simulink model "MPC"  (R2022b)
settings: Solver=VariableStepAuto  StartTime=0.0  StopTime=T_final*2  RelTol=1e-3
values from neighbouring files (symbols this model uses):
  Aineq = [zeros(n_int*L,n_states*(L+1)) eye(n_int*L) -eye(n_int*L) ... (first row only)    [Run_model.m]
  bineq = [kron(ones(L,1),u_up) ... (first row only)    [Run_model.m]
  d = 0.1    [Run_model.m]
  H = blkdiag(H1,H2,H3)    [Run_model.m]
  L = 10    [Run_model.m]    (also in encoder.m = 0.1175; measurement_model.m = 0.1175)
  n_int = 2    [Run_model.m]
  n_states = 3    [Run_model.m]
  Ts = 0.01    [Run_model.m]    (also in imu.m)
  z_initial = [theta0;x0;y0]    [Run_model.m]
settings Model: Creator=Abelb  LastModifiedBy=Abelb

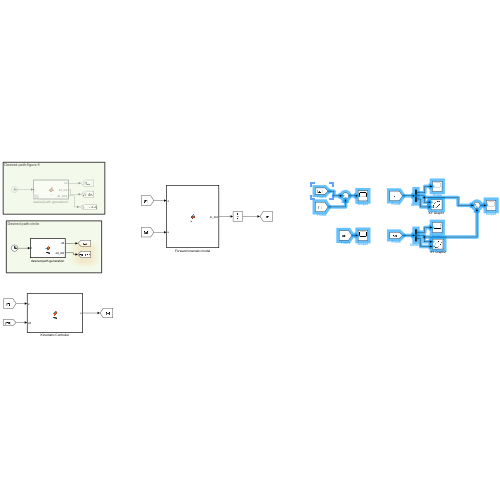
[thumbnail: Simulink's stored preview of the top-level diagram]
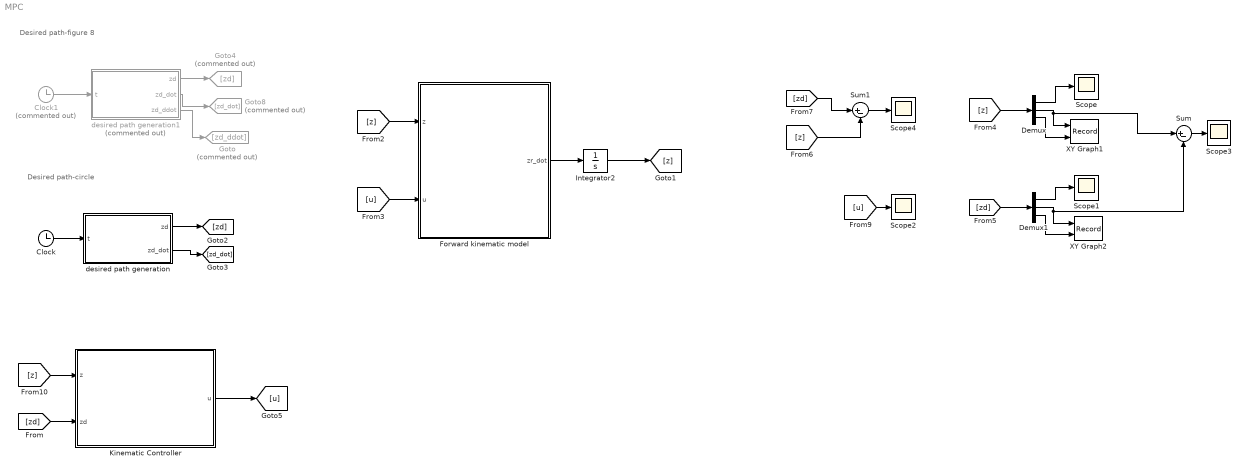
== system MPC ==
  note: Desired path-circle
  note: Desired path-figure 8
  Clock : Clock
  Clock1 : Clock  Commented=on
  Demux : Demux  Outputs=3
  Demux1 : Demux  Outputs=3
  Forward kinematic model : MATLAB Function  TreatAsAtomicUnit=on
  Goto : Goto  Commented=on  GotoTag=zd_ddot
  Goto4 : Goto  Commented=on  GotoTag=zd
  Goto8 : Goto  Commented=on  GotoTag=zd_dot
  Integrator2 : Integrator  InitialCondition=z_initial
  Kinematic Controller : MATLAB Function  TreatAsAtomicUnit=on
  Scope{,1..4} (5 alike) : Scope
  Sum : Sum  Inputs=|+-
  Sum1 : Sum  Inputs=|+-
  XY Graph1 : Record  FileSettingsInternal="{\"entries\":[{\"content\":{\"excelSettings\":{\"content\":{},\"type\":\"Streamout.ExcelSettings\"}},\"type\":\"Streamout.FileSettingStorage\",\"uuid\":\"ce67c0c4-7f67-4c88-aaae-392a4bc8995e\"}],\"packageUris\":[\"http://schema.mathworks.com/mf0/streamout_blocks/R2020a\"],\"version\":\"1.0\"}"  Layout=[1 1]  SignalsInternal="{\"entries\":[{\"content\":{\"signals\":[{\"content\":{\"blockPath\":[\"MPC/XY Graph1\"],\"channel\":[],\"dimensions\":[1],\"domain\":\"MPC/XY Graph1\",\"lineColor\":\"#a2142f\",\"plots\":[1],\"port\":1,\"sid\":[\"\"],\"signalID\":31603,\"signalName\":\"Demux:2\"},\"type\":\"RecordBlkView.Signal\",\"uuid\":\"af874ebe-007b-4861-a05c-edfc673b51a8\"},{\"content\":{\"blockPath\":[\"MPC/XY Graph1\"],\"channel\":[],\"dimensions\":[1],\"domain\":\"MPC/XY Graph1\",\"lineColor\":\"#139fff\",\"plots\":[1],\"port\":2,\"sid\":[\"\"],\"signalID\":31607,\"signalName\":\"Demux:3\"},\"type\":\"RecordBlkView.Signal\",\"uuid\":\"9c7c2835-5321-4135-b8aa-964658d863e7\"}]},\"type\":\"RecordBlkView.InputSignals\",\"uuid\":\"460cb3ef-f7a3-4bdc-882a-30f64cb38d6e\"}],\"packageUris\":[\"http://schema.mathworks.com/mf0/streamout_blocks/R2020a\"],\"version\":\"1.0\"}"  VisualizationBindings="{\"xyplotplugin\":{\"info\":[{\"series\":[{\"bindingParametersList\":[{\"parameter\":\"X-Axis\",\"signalID\":31603,\"signalName\":\"Demux:2\"},{\"parameter\":\"Y-Axis\",\"signalID\":31607,\"signalName\":\"Demux:3\"}],\"seriesID\":48364}],\"subplotID\":1}]}}"  CompatibilityTag=XY
  XY Graph2 : Record  FileSettingsInternal="{\"entries\":[{\"content\":{\"excelSettings\":{\"content\":{},\"type\":\"Streamout.ExcelSettings\"}},\"type\":\"Streamout.FileSettingStorage\",\"uuid\":\"94404df9-d188-4410-a8ad-29bdb399ae23\"}],\"packageUris\":[\"http://schema.mathworks.com/mf0/streamout_blocks/R2020a\"],\"version\":\"1.0\"}"  Layout=[1 1]  SignalsInternal="{\"entries\":[{\"content\":{\"signals\":[{\"content\":{\"blockPath\":[\"MPC/XY Graph2\"],\"channel\":[],\"dimensions\":[1],\"domain\":\"MPC/XY Graph2\",\"lineColor\":\"#a2142f\",\"plots\":[1],\"port\":1,\"sid\":[\"\"],\"signalID\":31611,\"signalName\":\"Demux1:2\"},\"type\":\"RecordBlkView.Signal\",\"uuid\":\"86dd43ab-7c69-451e-8692-9ec7fed00778\"},{\"content\":{\"blockPath\":[\"MPC/XY Graph2\"],\"channel\":[],\"dimensions\":[1],\"domain\":\"MPC/XY Graph2\",\"lineColor\":\"#139fff\",\"plots\":[1],\"port\":2,\"sid\":[\"\"],\"signalID\":31615,\"signalName\":\"Demux1:3\"},\"type\":\"RecordBlkView.Signal\",\"uuid\":\"e3c66422-9397-4330-95c8-babe7b5b194d\"}]},\"type\":\"RecordBlkView.InputSignals\",\"uuid\":\"cb7013a2-fe0a-4fd5-8dab-764f0a85911f\"}],\"packageUris\":[\"http://schema.mathworks.com/mf0/streamout_blocks/R2020a\"],\"version\":\"1.0\"}"  VisualizationBindings="{\"xyplotplugin\":{\"info\":[{\"series\":[{\"bindingParametersList\":[{\"parameter\":\"X-Axis\",\"signalID\":31611,\"signalName\":\"Demux1:2\"},{\"parameter\":\"Y-Axis\",\"signalID\":31615,\"signalName\":\"Demux1:3\"}],\"seriesID\":12711}],\"subplotID\":1}]}}"  CompatibilityTag=XY
  desired path generation : MATLAB Function  TreatAsAtomicUnit=on
  desired path generation1 : MATLAB Function  Commented=on  TreatAsAtomicUnit=on
  wires:
  Forward kinematic model/1(zr_dot) -> Integrator2/1
  desired path generation1/3(zd_ddot) -> Goto/1
  Clock1/1 -> desired path generation1/1(t)
  desired path generation1/2(zd_dot) -> Goto8/1
  desired path generation1/1(zd) -> Goto4/1
  desired path generation/2(zd_dot) -> [zd_dot]
  desired path generation/1(zd) -> [zd]
  Clock/1 -> desired path generation/1(t)
  [zd] -> Kinematic Controller/2(zd)
  Integrator2/1 -> [z]
  [z] -> Forward kinematic model/1(z)
  [z] -> Demux/1
  Demux/1 -> Scope/1
  Demux/2 -> XY Graph1/1, Sum/1
  Demux/3 -> XY Graph1/2
  Demux1/2 -> XY Graph2/1, Sum/2
  Demux1/3 -> XY Graph2/2
  [zd] -> Demux1/1
  Demux1/1 -> Scope1/1
  Sum/1 -> Scope3/1
  Kinematic Controller/1(u) -> [u]
  [zd] -> Sum1/1
  [z] -> Sum1/2
  Sum1/1 -> Scope4/1
  [u] -> Scope2/1
  [u] -> Forward kinematic model/2(u)
  [z] -> Kinematic Controller/1(z)

== matlab function MPC/desired path generation1 ==
  data: t input; zd output; zd_dot output; zd_ddot output
function [zd,zd_dot,zd_ddot] = fcn(t)

t = t/50;

a=1;
x = a*cos(t)/(1+sin(t)^2);
y = a*sin(t)*cos(t)/(1+sin(t)^2);
% unit circle (radius = 1; origin: (0,0))
zd = [atan(y./x);              % theta
      a*cos(t)/(1+sin(t)^2);         % x
      a*sin(t)*cos(t)/(1+sin(t)^2)];        % y

zd_dot = [ 0;
          -a*sin(t)*(cos(t)^2+2)/(1+sin(t)^2)^2;
          (a*cos(t)^2-2*a*sin(t)^2)/(1+sin(t)^2)^2];

z1 = (a*sin(t)^2*cos(t)^3-11*a*cos(t)^3+8*a*cos(t))/(1+sin(t)^2)^3;
z2 = -2*a*sin(t)*cos(t)*(3+2*cos(t)^2-sin(t)^2)/(1+sin(t)^2)^3;
zd_ddot = [z1;
           z2];

== matlab function MPC/Kinematic Controller ==
  data: z input; u output; zd input; Aineq parameter; bineq parameter; L parameter; n_states parameter; n_int parameter; Ts parameter; d parameter; H parameter
function u = fcn(z,zd,Aineq,bineq,L,n_states, n_int,Ts,d, H)

%% unpacking inputs
% theta = z(1);
% x = z(2);
% y = z(3);
% xd = zd(2);
% yd = zd(3);
% xd_dot = zd_dot(2);
% yd_dot = zd_dot(3);

zd = [zd(1);
      zd(2);
      zd(3)];
z_full = zeros(n_states*(L+1)+n_int*2*L,1);

%% controller
% K1 = [cos(theta) sin(theta);
%      -sin(theta)/d cos(theta)/d];
% K2 = [xd_dot + kx*sin( atan( kx*(xd-x) ) );
%       yd_dot + ky*sin( atan( ky*(yd-y) ) )];
% u = K1*K2;

coder.extrinsic("MPC_controller");
z_full(:) = MPC_controller(z,zd,H,Aineq,bineq,L,n_states, n_int,Ts,d);

% D_bar = @(N,n)[zeros((N-1)*n,n), eye((N-1)*n)];
% D_under = @(N,n)[eye((N-1)*n),zeros((N-1)*n,n)];
% E = kron([1, zeros(1,L)],eye(n_states));
% A = @(z) [1 0 0;
%      -Ts*sin(z(1))-d*Ts*cos(z(1)) 1 0;
%      Ts*cos(z(1))-d*Ts*sin(z(1)) 0 1];
% B = @(z) Ts*[0 1;
%           cos(z(1)) -d*sin(z(1));
%           sin(z(1)) d*cos(z(1))];
% Aeq = @(z) [D_bar(L+1,n_states)-kron(eye(L),A(z))*D_under(L+1,n_states) -kron(eye(L),B(z)) zeros(L*n_states,n_int*L);
%             E zeros(n_states,n_int*L) zeros(n_states,n_int*L)];
% beq = [zeros(L*n_states,1); z];
% 
% z_full(:) = quadprog(H,zeros(size(z_full,1),1),Aineq,bineq,Aeq(zd),beq);



%% packing output
u = z_full((L+1)*n_states+1:(L+1)*n_states+n_int);

== matlab function MPC/Forward kinematic model ==
  data: z input; u input; zr_dot output; d parameter
function zr_dot = fcn(z,u,d)

%% unpacking the state vectors
theta=z(1);

%% unpacking the intput
v=u(1);
omega=u(2);

%% ODE
theta_dot=omega;
x_dot=v*cos(theta)-d*omega*sin(theta);
y_dot=v*sin(theta)+d*omega*cos(theta);
% phir_dot = (v+omega)/r;
% phil_dot = (v-omega)/r;


%% packing the output
zr_dot=[theta_dot;x_dot;y_dot];

== matlab function MPC/desired path generation ==
  data: t input; zd output; zd_dot output
function [zd,zd_dot] = fcn(t)

 t = t/150;


% unit circle (radius = 1; origin: (0,0))
zd = [t;
      sin(2*t);         % x
      1-1*cos(2*t)];        % y

zd_dot = [1;
          2*cos(2*t);
          2*sin(2*t)];
